simulink model "Problem_1week2"  (R2020a)
settings: Solver=VariableStepAuto  StartTime=0.0  StopTime=10.0  RelTol=1e-3
settings Model: Creator=hp  LastModifiedBy=hp

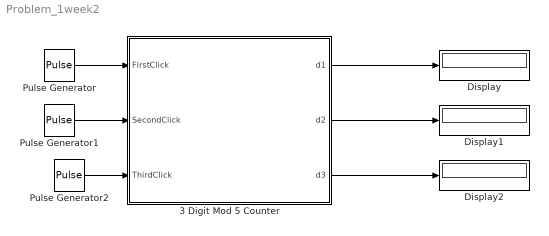
== system Problem_1week2 ==
  3 Digit Mod 5 Counter : Stateflow chart  TreatAsAtomicUnit=on
  Display : Display
  Display1 : Display
  Display2 : Display
  Pulse Generator : DiscretePulseGenerator  PulseType=Time based  Period=10  PulseWidth=5
  Pulse Generator1 : DiscretePulseGenerator  PulseType=Time based  Period=10  PulseWidth=5
  Pulse Generator2 : DiscretePulseGenerator  PulseType=Time based  Period=10  PulseWidth=5
  wires:
  3 Digit Mod 5 Counter/1(d1) -> Display/1
  3 Digit Mod 5 Counter/2(d2) -> Display1/1
  3 Digit Mod 5 Counter/3(d3) -> Display2/1
  Pulse Generator2/1 -> 3 Digit Mod 5 Counter/3(ThirdClick)
  Pulse Generator1/1 -> 3 Digit Mod 5 Counter/2(SecondClick)
  Pulse Generator/1 -> 3 Digit Mod 5 Counter/1(FirstClick)

== stateflow chart Problem_1week2/3 Digit Mod 5 Counter ==
  state DigitTwo
    state One
      en:
      d2=1;
    state Two
      en:
      d2=2;
    state Zero
      en:
      d2=0;
    state Four
      en:
      d2=4;
    state Three
      en:
      d2=3;
    DigitTwo.Two -> DigitTwo.Three : [SecondClick]
    DigitTwo.Zero -> DigitTwo.One : [SecondClick]
    DigitTwo.One -> DigitTwo.Two : [SecondClick]
    (default) -> DigitTwo.Zero
    DigitTwo.Four -> DigitTwo.Zero : [SecondClick]/{ThirdClick}
    DigitTwo.Three -> DigitTwo.Four : [SecondClick]
  state DigitOne
    state One
      en:
      d1=1;
    state Two
      en:
      d1=2;
    state Zero
      en:
      d1=0;
    state Three
      en:
      d1=3;
    state Four
      en:
      d1=4;
    DigitOne.Zero -> DigitOne.One : [FirstClick]
    DigitOne.One -> DigitOne.Two : [FirstClick]
    DigitOne.Two -> DigitOne.Three : [FirstClick]
    (default) -> DigitOne.Zero
    DigitOne.Four -> DigitOne.Zero : [FirstClick]/{SecondClick}
    DigitOne.Three -> DigitOne.Four : [FirstClick]
  state DigitThree
    state One
      en:
      d3=1;
    state Two
      en:
      d3=2;
    state Zero
      en:
      d3=0;
    state Three
      en:
      d3=3;
    state Four
      en:
      d3=4;
    DigitThree.Two -> DigitThree.Three : [ThirdClick]
    DigitThree.Zero -> DigitThree.One : [ThirdClick]
    DigitThree.One -> DigitThree.Two : [ThirdClick]
    (default) -> DigitThree.Zero
    DigitThree.Four -> DigitThree.Zero : [ThirdClick]
    DigitThree.Three -> DigitThree.Four : [ThirdClick]
  (default) -> DigitOne
  data: d1 output; d2 output; d3 output; FirstClick input; SecondClick input; ThirdClick input
